simulink model "model_lat_SAS"  (R2024a)
settings: Solver=VariableStepAuto  StartTime=0.0  StopTime=20.0  MaxStep=0.1  RelTol=1e-3
values from neighbouring files (symbols this model uses):
  Kbetadr = get_feedback_gain(sysLatAugClosedLoop('sideslip angle', 'rudder'),      0.7, 'Dutch roll', 0.01, 1.0)    [task3.m]
  Kphida = 0.2    [task3.m]
  Krdr = get_feedback_gain(-sysLatAug('washed out yaw rate', 'rudder'),      0.7, 'Dutch roll', 0.5, 1.5)    [task3.m]
  sysLat = ss(Alat, Blat, Clat, Dlat)    [model_lat.m]
  washoutFilter = tf([timeConstant, 0], [timeConstant, 1])    [generate_washout_filter.m]    (also in task3.m = generate_washout_filter(tauWashoutFilter))
settings Model: Creator=hnamtang  LastModifiedBy=hnamtang

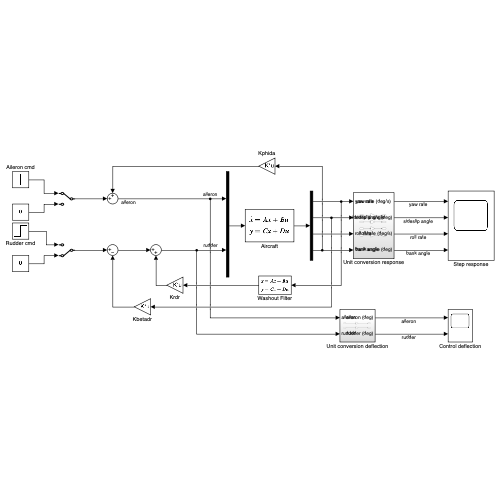
[thumbnail: Simulink's stored preview of the top-level diagram]
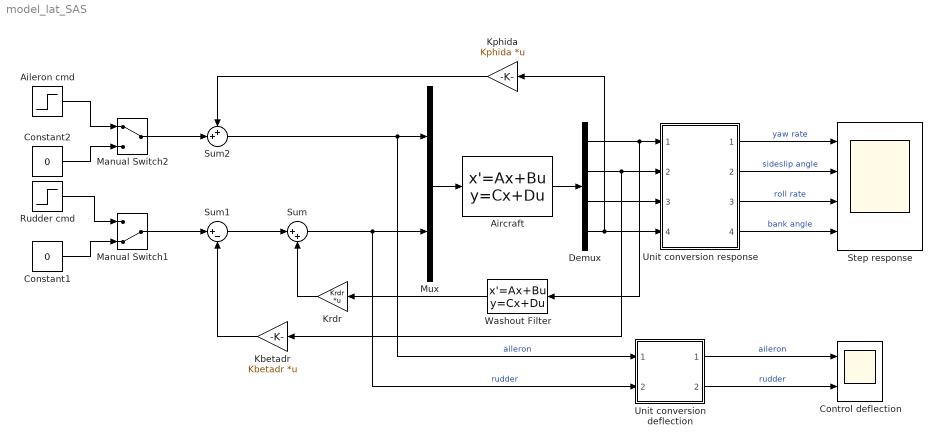
== system model_lat_SAS ==
  Aileron cmd : Step  After=deg2rad(20)  SampleTime=0
  Aircraft : StateSpace  A=sysLat.A  B=sysLat.B  C=sysLat.C  D=sysLat.D  InitialCondition=0
  Constant1 : Constant  Value=0
  Constant2 : Constant  Value=0
  Control deflection : Scope  NumInputPorts=2
  Demux : Demux
  Kbetadr : Gain  Gain=Kbetadr  Multiplication=Matrix(K*u)
  Kphida : Gain  Gain=Kphida  Multiplication=Matrix(K*u)
  Krdr : Gain  Gain=Krdr  Multiplication=Matrix(K*u)
  Manual Switch1 : ManualSwitch  CurrentSetting=0
  Manual Switch2 : ManualSwitch
  Mux : Mux  Inputs=2
  Rudder cmd : Step  After=deg2rad(20)  SampleTime=0
  Step response : Scope  NumInputPorts=4
  Sum : Sum  Inputs=|++
  Sum1 : Sum  Inputs=|+-
  Sum2 : Sum  Inputs=++|
  Unit conversion deflection : Subsystem
  Unit conversion response : Subsystem
  Washout Filter : StateSpace  A=washoutFilter.A  B=washoutFilter.B  C=washoutFilter.C  D=washoutFilter.D  InitialCondition=0
  wires:
  Demux/4 -> Unit conversion response/4(bank angle), Kphida/1
  Aircraft/1 -> Demux/1
  Demux/1 -> Unit conversion response/1(yaw rate), Washout Filter/1
  Mux/1 -> Aircraft/1
  Sum2/1 -> Mux/1, Unit conversion deflection/1(aileron)  "aileron"
  Washout Filter/1 -> Krdr/1
  Krdr/1 -> Sum/2
  Demux/2 -> Unit conversion response/2(sideslip angle), Kbetadr/1
  Sum1/1 -> Sum/1
  Kbetadr/1 -> Sum1/2
  Kphida/1 -> Sum2/1
  Sum/1 -> Mux/2, Unit conversion deflection/2(rudder)  "rudder"
  Manual Switch1/1 -> Sum1/1
  Rudder cmd/1 -> Manual Switch1/1
  Constant1/1 -> Manual Switch1/2
  Constant2/1 -> Manual Switch2/2
  Aileron cmd/1 -> Manual Switch2/1
  Manual Switch2/1 -> Sum2/2
  Demux/3 -> Unit conversion response/3(roll rate)
  Unit conversion response/1("yaw rate (deg/s) ") -> Step response/1  "yaw rate"
  Unit conversion response/2(sideslip angle (deg)) -> Step response/2  "sideslip angle"
  Unit conversion response/3(roll rate (deg/s)) -> Step response/3  "roll rate"
  Unit conversion response/4(bank angle (deg)) -> Step response/4  "bank angle"
  Unit conversion deflection/1(aileron (deg)) -> Control deflection/1  "aileron"
  Unit conversion deflection/2(rudder (deg)) -> Control deflection/2  "rudder"

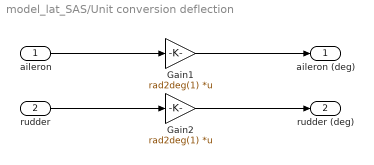
== system model_lat_SAS/Unit conversion deflection ==
  aileron : Inport
  rudder : Inport  Port=2
  Gain1 : Gain  Gain=rad2deg(1)  Multiplication=Matrix(K*u)
  Gain2 : Gain  Gain=rad2deg(1)  Multiplication=Matrix(K*u)
  aileron (deg) : Outport
  rudder (deg) : Outport  Port=2
  wires:
  Gain2/1 -> rudder (deg)/1
  aileron/1 -> Gain1/1
  rudder/1 -> Gain2/1
  Gain1/1 -> aileron (deg)/1

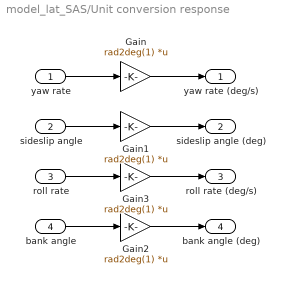
== system model_lat_SAS/Unit conversion response ==
  yaw rate : Inport
  sideslip angle : Inport  Port=2
  roll rate : Inport  Port=3
  bank angle : Inport  Port=4
  Gain{,1..3} (4 alike) : Gain  Gain=rad2deg(1)  Multiplication=Matrix(K*u)
  "yaw rate (deg/s) " : Outport
  sideslip angle (deg) : Outport  Port=2
  roll rate (deg/s) : Outport  Port=3
  bank angle (deg) : Outport  Port=4
  wires:
  bank angle/1 -> Gain2/1
  roll rate/1 -> Gain3/1
  yaw rate/1 -> Gain/1
  Gain/1 -> "yaw rate (deg/s) "/1
  sideslip angle/1 -> Gain1/1
  Gain1/1 -> sideslip angle (deg)/1
  Gain3/1 -> roll rate (deg/s)/1
  Gain2/1 -> bank angle (deg)/1
